simulink model "SIMULAZIONE"  (R2023a)
settings: Solver=VariableStepAuto  StartTime=0.0  StopTime=10.0  RelTol=1e-3
values from neighbouring files (symbols this model uses):
  K_fb = K(1:1,1:4)    [TRACKING.m]
  K_ff = K(1:1,5:6)    [TRACKING.m]
  parametri = [m; Iz; Lf; Lr; Cf; Cr; Vx]    [TRACKING.m]
  Vx = 10    [TRACKING.m]    (also in bicycle.m = block.DialogPrm(2).Data(7))
  X0 = data_scenario1.data.ActorSpecifications(1,1).Position(1)    [TRACKING.m]    (also in sim_data.mat = -2.8)
  x_0 = [0 0 yaw_0 0]    [TRACKING.m]
  Y0 = data_scenario1.data.ActorSpecifications(1,1).Position(2)    [TRACKING.m]    (also in sim_data.mat = 6.6)
undefined symbols (not defined in the file or in its folder): sigbuilder_block
libraries: drivingscenarioandsensors x1
settings Model: Creator=Randy  LastModifiedBy=Randy

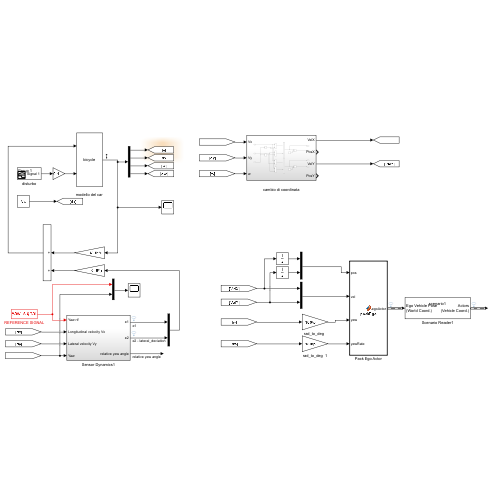
[thumbnail: Simulink's stored preview of the top-level diagram]
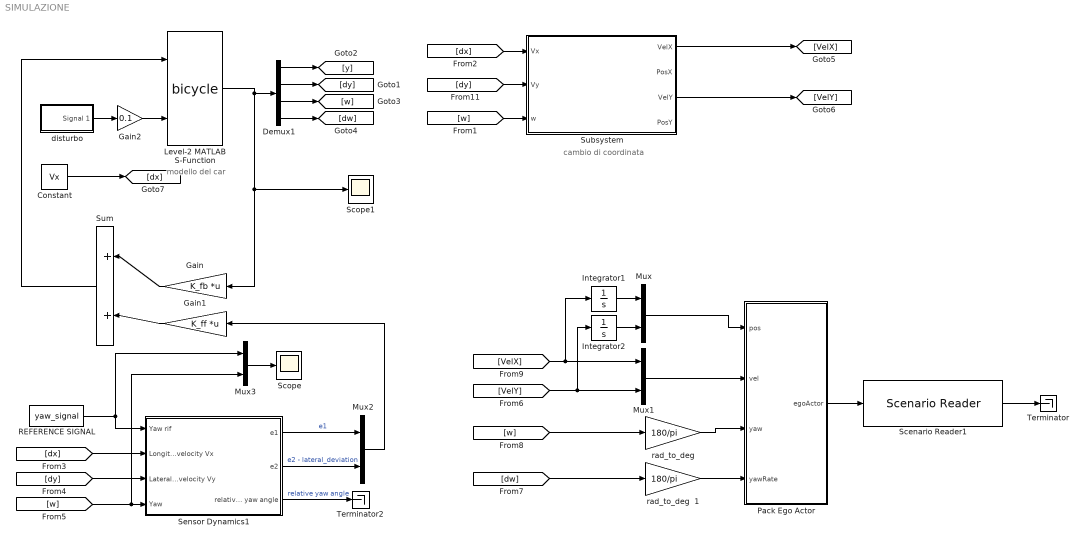
== system SIMULAZIONE ==
  note: cambio di coordinata
  note: modello del car
  Constant : Constant  Value=Vx
  Demux1 : Demux
  Gain : Gain  Gain=K_fb  Multiplication=Matrix(K*u)
  Gain1 : Gain  Gain=K_ff  Multiplication=Matrix(K*u)
  Gain2 : Gain  Gain=0.1
  Integrator1 : Integrator  InitialCondition=0.05
  Integrator2 : Integrator  InitialCondition=0.05
  Level-2 MATLAB S-Function : M-S-Function  FunctionName=bicycle  Parameters=x_0,parametri
  Mux{,1..3} (4 alike) : Mux  Inputs=2
  Pack Ego Actor : MATLAB Function  TreatAsAtomicUnit=on
  REFERENCE SIGNAL : FromWorkspace  VariableName=yaw_signal  OutputAfterFinalValue=Holding final value
  Scenario Reader1 : drivingscenarioandsensors/Scenario Reader  ScenarioSource=From file  ScenarioFileName=C:\Users\Randy\Documents\secondo modulo\scenario1.mat  ScenarioVariableName=scenario  OutputCoordinateSystem=Vehicle coordinates  EgoVehicleSource=Input port  EgoVehicleActorID=1  OrientVehiclesOnRoad=off  OutputEgoVehiclePose=on  OutputEgoVehicleState=off  SampleTime=0.1  LaneBoundaryOutput=None  LaneBoundaryDistance=0:0.5:9.5  LaneBoundaryLocation=Center of lane markings  BusNameSource=Auto  BusName=BusActors  BusNumActorsSource=Scenario  BusNumActors=100  BusName2Source=Auto  BusName2=BusLaneBoundaries  BusNumLaneBoundariesSource=Scenario  BusNumLaneBoundaries=10  BusName3Source=Auto  BusName3=BusEgoActor  BusName4Source=Auto  BusName4=BusEgoState  ShowCoordinateLabels=on  SimulateUsing=Interpreted execution
  Scope : Scope
  Scope1 : Scope
  Sensor Dynamics1 : Subsystem
  Subsystem : Subsystem
  Sum : Sum  Inputs=|++
  Terminator : Terminator
  Terminator2 : Terminator
  disturbo : Subsystem  Tag=STV Subsys  LoadFcn=sigbuilder_block('load');  StartFcn=sigbuilder_block('start');  StopFcn=sigbuilder_block('stop');  ClipboardFcn=sigbuilder_block('clipboard');  mask(Sigbuilder block){tuvar=[0:10]}
      mask help: Simulink:masks:SigbuilderBlock_MD
      mask init:
      | if ~strcmp(get_param(bdroot(gcbh),'SimulationStatus'),'stopped') tuvar = sigbuilder_block('maskInit'); end
      settings: CopyFcn=sigbuilder_block('copy');  DeleteFcn=sigbuilder_block('delete');  ModelCloseFcn=sigbuilder_block('modelClose');  PreSaveFcn=sigbuilder_block('preSave');  PauseFcn=sigbuilder_block('pause');  ContinueFcn=sigbuilder_block('continue');  NameChangeFcn=sigbuilder_block('namechange');  OpenFcn=sigbuilder_block('open',[5.4 5.4 1141.2 580.8 ]);  CloseFcn=sigbuilder_block('close');
      mask Display: plot(0, 0, 100, 100,[2, 2, 32, 32, 2], [68, 8, 8, 68, 68],[32, 2], [38, 38], [32, 19, 2],[53, 60, 44], [32, 17, 17, 2],[16, 16, 31, 31]);txt = getActiveGroup(gcbh);text(2, 100, txt,'verticalAlignment', 'top');
  "rad_to_deg  " : Gain  Gain=180/pi
  rad_to_deg  1 : Gain  Gain=180/pi
  wires:
  [w] -> "rad_to_deg  "/1
  [w] -> Subsystem/3(w)
  [w] -> Mux3/2, Sensor Dynamics1/4("Yaw ")
  Sensor Dynamics1/3(relative yaw angle) -> Terminator2/1  "relative yaw angle"
  REFERENCE SIGNAL/1 -> Mux3/1, Sensor Dynamics1/1(Yaw rif)
  Pack Ego Actor/1(egoActor) -> Scenario Reader1/1
  rad_to_deg  1/1 -> Pack Ego Actor/4(yawRate)
  "rad_to_deg  "/1 -> Pack Ego Actor/3(yaw)
  Integrator2/1 -> Mux/2
  Subsystem/1(VelX) -> [VelX]
  [dw] -> rad_to_deg  1/1
  Gain/1 -> Sum/1
  Mux2/1 -> Gain1/1
  Scenario Reader1/1 -> Terminator/1
  [VelX] -> Mux1/1, Integrator1/1
  [VelY] -> Mux1/2, Integrator2/1
  [dx] -> Sensor Dynamics1/2(Longitudinal velocity Vx)
  Sum/1 -> Level-2 MATLAB S-Function/1
  Constant/1 -> [dx]
  Mux1/1 -> Pack Ego Actor/2(vel)
  Mux/1 -> Pack Ego Actor/1(pos)
  Integrator1/1 -> Mux/1
  Demux1/3 -> [w]
  Gain2/1 -> Level-2 MATLAB S-Function/2
  Sensor Dynamics1/2(e2) -> Mux2/2  "e2 - lateral_deviation"
  Mux3/1 -> Scope/1
  [dx] -> Subsystem/1(Vx)
  disturbo/1(Signal 1) -> Gain2/1
  Subsystem/3(VelY) -> [VelY]
  Level-2 MATLAB S-Function/1 -> Scope1/1, Gain/1, Demux1/1
  Gain1/1 -> Sum/2
  Sensor Dynamics1/1(e1) -> Mux2/1  "e1"
  Demux1/1 -> [y]
  [dy] -> Subsystem/2(Vy)
  Demux1/2 -> [dy]
  [dy] -> Sensor Dynamics1/3(Lateral velocity Vy)
  Demux1/4 -> [dw]

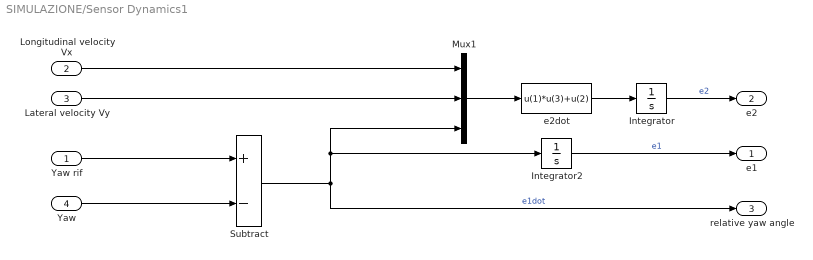
== system SIMULAZIONE/Sensor Dynamics1 ==
  Yaw rif : Inport
  Longitudinal velocity Vx : Inport  Port=2
  Lateral velocity Vy : Inport  Port=3
  "Yaw " : Inport  Port=4
  Integrator : Integrator
  Integrator2 : Integrator
  Mux1 : Mux  Inputs=[1 1 1]
  Subtract : Sum  Inputs=+-
  e2dot : Fcn  Expr=u(1)*u(3)+u(2)
  e1 : Outport  VectorParamsAs1DForOutWhenUnconnected=off
  e2 : Outport  Port=2  VectorParamsAs1DForOutWhenUnconnected=off
  relative yaw angle : Outport  Port=3  VectorParamsAs1DForOutWhenUnconnected=off
  wires:
  Integrator2/1 -> e1/1  "e1"
  Mux1/1 -> e2dot/1
  e2dot/1 -> Integrator/1
  Longitudinal velocity Vx/1 -> Mux1/1
  Lateral velocity Vy/1 -> Mux1/2
  Integrator/1 -> e2/1  "e2"
  Yaw rif/1 -> Subtract/1
  "Yaw "/1 -> Subtract/2
  Subtract/1 -> Integrator2/1, Mux1/3, relative yaw angle/1  "e1dot"

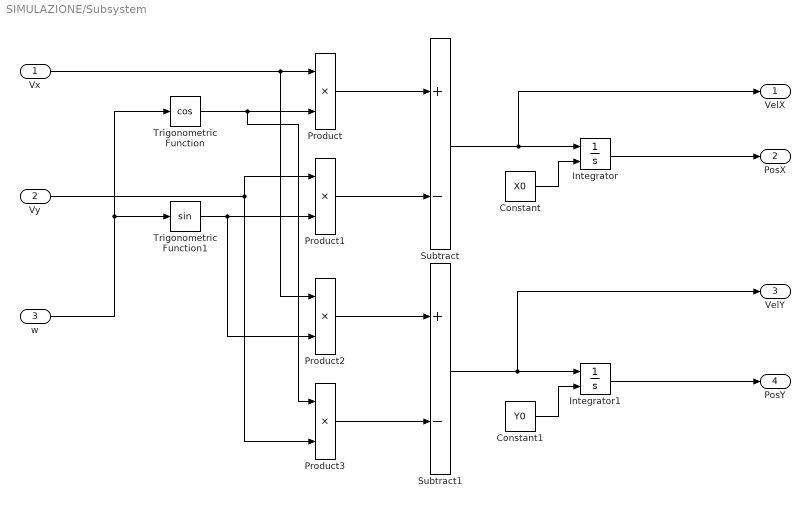
== system SIMULAZIONE/Subsystem ==
  Vx : Inport
  Vy : Inport  Port=2
  w : Inport  Port=3
  Constant : Constant  Value=X0
  Constant1 : Constant  Value=Y0
  Integrator : Integrator  InitialConditionSource=external
  Integrator1 : Integrator  InitialConditionSource=external
  Product{,1..3} (4 alike) : Product
  Subtract : Sum  Inputs=+-
  Subtract1 : Sum  Inputs=+-
  Trigonometric Function : Trigonometry  Operator=cos
  Trigonometric Function1 : Trigonometry
  VelX : Outport
  PosX : Outport  Port=2
  VelY : Outport  Port=3
  PosY : Outport  Port=4
  wires:
  Vx/1 -> Product2/1, Product/1
  w/1 -> Trigonometric Function1/1, Trigonometric Function/1
  Trigonometric Function/1 -> Product3/1, Product/2
  Trigonometric Function1/1 -> Product2/2, Product1/2
  Product1/1 -> Subtract/2
  Product/1 -> Subtract/1
  Subtract/1 -> VelX/1, Integrator/1
  Integrator/1 -> PosX/1
  Constant/1 -> Integrator/2
  Product2/1 -> Subtract1/1
  Product3/1 -> Subtract1/2
  Subtract1/1 -> VelY/1, Integrator1/1
  Constant1/1 -> Integrator1/2
  Integrator1/1 -> PosY/1
  Vy/1 -> Product3/2, Product1/1

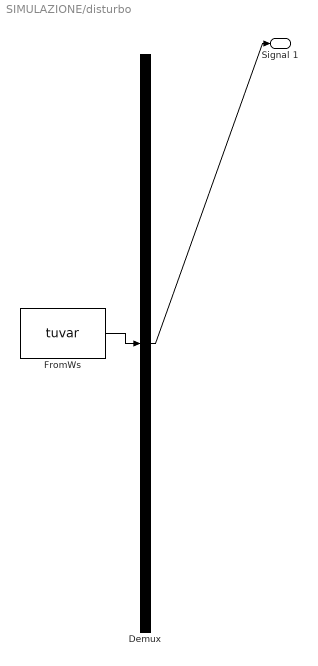
== system SIMULAZIONE/disturbo ==
  Demux : Demux  Tag=STV Demux  Outputs=1
      settings: DisplayOption=none
  FromWs : FromWorkspace  Tag=STV FromWs  VariableName=tuvar
      SigBuilderData=|
      | common.afterFinalStr = 'Extrapolate'
      | common.sampleTime = 0
      | dataSet.timeRange = [0 10]
      | dataSet.name = 'Group 1'
      | sbobj.Groups.Name = 'Group 1'
      | sbobj.Groups.Signals.Name = 'Signal 1'
      | sbobj.Groups.Signals.XData = [0 0.105263157895 0.210526315789 0.315789473684 0.421052631579 0.526315789474 0.631578947368 0.736842105263 0.842105263158 0.947368421053 1.05263157895 1.15789473684 1.26315789474 1.36842105263 1.47368421053 1.57894736842 1.68421052632 1.78947368421 1.89473684211 2 2.10526315789 2.21052631579 2.31578947368 2.42105263158 2.52631578947 2.63157894737 2.73684210526 2.84210526316 2.94736842105 3.05263157895 3.15789473684 3.26315789474 3.36842105263 3.47368421053 3.57894736842 3.68421052632 3.78947368421 3.89473684211 4 4.10526315789 4.21052631579 4.31578947368 4.42105263158 4.52631578947 4.63157894737 4.73684210526 4.84210526316 4.94736842105 5.05263157895 5.15789473684 5.26315789474 5.36842105263 5.47368421053 5.57894736842 5.68421052632 5.78947368421 5.89473684211 6 6.10526315789 6.21052631579 6.31578947368 6.42105263158 6.52631578947 6.63157894737 6.73684210526 6.84210526316 6.94736842105 7.05263157895 7.15789473684 7.26315789474 7.36842105263 7.47368421053 7.57894736842 7.68421052632 7.78947368421 7.89473684211 8 8.10526315789 8.21052631579 8.31578947368 8.42105263158 8.52631578947 8.63157894737 8.73684210526 8.84210526316 8.94736842105 9.05263157895 9.15789473684 9.26315789474 9.36842105263 9.47368421053 9.57894736842 9.68421052632 9.78947368421 9.89473684211 10]
      | sbobj.Groups.Signals.YData = [0 0 0 0 0 0 0 0 0 0 0 0 0 0 0 0 0 0 0 0 0 0 0 0 0 0 0 0 0 0 0 0 0 0 0 0 0 0 0 0.324699469205 0.61421271269 0.837166478263 0.969400265939 0.996584493007 0.915773326655 0.735723910673 0.475947393037 0.164594590281 -0.164594590281 -0.475947393037 -0.735723910673 -0.915773326655 -0.996584493007 -0.969400265939 -0.837166478263 -0.61421271269 -0.324699469205 0 0 0 0 0 0 0 0 0 0 0 0 0 0 0 0 0 0 0 0 0 0 0 0 0 0 0 0 0 0 0 0 0 0 0 0 0 0 0]
  Signal 1 : Outport  Tag=STV Outport
  wires:
  Demux/1 -> Signal 1/1
  FromWs/1 -> Demux/1

== matlab function SIMULAZIONE/Pack Ego Actor ==
  data: pos input; egoActor output Bus: BusActors1Actors size=1; vel input; yaw input; yawRate input
function egoActor = packEgo(pos,vel,yaw,yawRate)
% Pack ego information into a single ego actor bus
%
% Imoprtant note:
% Output is a bus of type BusActorsActors. This is the same bus used by the
% Scenario Reader to output an individual actor. If you change the
% output bus name of Scenario Reader, change the output bus name here
% as well by clicking on 'Edit Data' in the menu above.

%Position x,y,z
%Velocity x,y,z
%Angular velocity wx, wy, wz

egoActor = struct(...
    'ActorID',1,...
    'Position', [pos(1) pos(2) 0], ...
    'Velocity', [vel(1) vel(2) 0], ...
    'Roll', 0, ...
    'Pitch', 0, ...
    'Yaw', yaw, ...
    'AngularVelocity', [0 0 yawRate]);
